simulink model "FIC_hapticControl"  (R2019b)
settings: Solver=VariableStepAuto  StartTime=0.0  StopTime=inf  FixedStep=0.00001
model workspace: external: MATLAB File /home/sydney/Desktop/matlab/simulink/SimpImpCheck/Assembly1_DataFile.m (data not in the file)
undefined symbols (not defined in the file or in its folder): smiData, X, Y, Z
libraries: sm_lib x21, nesl_utility x17, fl_lib x16, ee_lib x3
(part 2 of 2)

== matlab function FIC_hapticControl/Subsystem/MATLAB Function1 ==
  data: dxd input; Xd input; Fdes input; Wmax input; x0 input; xb input; K0 input; F input; DXd output; Wmax output; x0 output; xb output; K0 output; X input
function [DXd,Wmax,x0,xb,K0] = FICDx(dxd,Xd,Fdes,Wmax,x0,xb,K0, F,X)
% b damping - /20?
haptic=false;
if haptic
b=(xb-x0)/20;
% K0 Stiffness 
if K0>=(Wmax/x0)
    % Wmax - max torque/wrench
   K0=(Wmax/x0);
end

% Force = stiffness * displacement for the end effector? last section?
% About the spring section? B and 0?
F0=K0*x0;
% end effector desired position derivative - end effector desired velocity. 
% 
dx0d=Fdes/K0;
%When desired linear reaches 1% of end effector desired velocity 
dx0=0.01*dx0d;
% Force currently being applied is not equal to desired force
% haptic search of contact
if F~=Fdes && F~= 0
    % if current position is less than desired position
    if abs(X)<=abs(Xd)
        % Velocity = desired position + dx0d? what is this x0d
        DXd=Xd+dx0d;
    else
        % change in x = (Fdesired - currentF) * 0.01 * desired pose linear region/ desired
        % force. 
        dx=(Fdes-F)*dx0/Fdes;
        % Desired Pose = desired pose + a small change in desired pose 
        DXd=dxd+dx;
    end
else
    DXd=dxd;  
end
else
    DXd=Xd;
end

end







% if F~=Fdes
%     % %          if abs(Fdes)<=F0
%     % %              DXd=Xd+(X-Xd)*Fdes/((X-Xd)*K0+(F-Fdes));
%     if F~=0
%         DXdf=((X-Xd)*Fdes)/(F);
%         if DXdf>xb
%             DXd=Fdes/K0+sign(Fdes)*xb;
%         else
%             DXd=Fdes/K0-((X-Xd)*Fdes)/(F);
%         end
%     else
%         DXd=Fdes/K0+dxd;
%     end
%     % % else
%     % %     DXd=Xd+Wmax/((F-Wmax)/(X-Xd));
%     % % end
%     if DXd>xb
%         DXd=xb;
%     end
% else
%     DXd=dxd;
% end

% 
% function [DXd,Wmax,x0,xb,K0] = FICDx(dxd,Xd,Fdes,Wmax,x0,xb,K0,F,X)
% % b damping - /20?
% b=(xb-x0)/20;
% % K0 Stiffness 
% if K0>=(Wmax/x0)
%     % Wmax - max torque/wrench
%    K0=(Wmax/x0);
% end
% 
% % Force = stiffness * displacement for the end effector? last section?
% % About the spring section? B and 0?
% F0=K0*x0;
% % end effector desired position derivative - end effector desired velocity. 
% % 
% dx0d=Fdes/K0;
% % dividing desired by 100?
% dx0=0.01*dx0d;
% % Force currently being applied is not equal to desired force
% if F~=Fdes
%     % if current position is less than desired position
%     if abs(X)<=abs(Xd)
%         % Velocity = desired position + 
%         DXd=Xd+dx0d;
%     else
%         %DXd=dxd+sign(Fdes-F)*dx;
%         dx=(Fdes-F)*dx0/Fdes;
%         DXd=dxd+dx;
% 
%     end
% else
%     DXd=dxd;  
% end
% end

== matlab function FIC_hapticControl/Subsystem1/MATLAB Function ==
  data: xmax output; Xmax input; F output; dx input; x input; Wmax input; x0 input; xb input; K0 input
function [xmax,F]=fractalImpedenceControlFc(Xmax,dx,x,Wmax,x0,xb,K0)
b=(xb-x0)/20;
if sign(x)==-sign(dx) || abs(dx)<10^(-4)
    xmax=x;
    AbsErr=abs(x);
    if AbsErr<x0
        F=K0*x;
    else
        F=sign(x)*((1-exp(-abs(AbsErr - x0)./b)).*...
            (Wmax - K0.*x0)+K0.*x0);
    end
else
    if Xmax==0 || x>Xmax
        xmax=x;
    else
        xmax=Xmax;
        
    end
    xmid=xmax/2;
    AbsXmax=abs(xmax);
    if AbsXmax<x0
        Fmax=K0*xmax;
    else
        Fmax=sign(xmax)*((1-exp(-abs(AbsXmax - x0)./b)).*...
            (Wmax - K0.*x0)+K0.*x0);
    end
    Kout=Fmax/abs(xmid);
    F=-Kout*(xmid-x);
end

end

== matlab function FIC_hapticControl/MATLAB Function5 ==
  data: angles input; xPos output; dimensions input; yPos output; zPos output
function [xPos, yPos, zPos]  = FK(angles, dimensions)

ang1 = angles(1);
ang2 = angles(2);
ang3 = angles(3);
L1 = dimensions(1);
L2 = dimensions(2);
L3 = dimensions(3);

xPos = (L1*cos(ang1) + L2*cos(ang1 + ang2) + L3*cos(ang1 + ang2 + ang3));
yPos = (L1*sin(ang1) + L2*sin(ang1 + ang2) + L3*sin(ang1 + ang2 + ang3));
zPos = 0;

== matlab function FIC_hapticControl/Subsystem1/MATLAB Function1 ==
  data: dxd input; Xd input; Fdes input; Wmax input; x0 input; xb input; K0 input; F input; DXd output; Wmax output; x0 output; xb output; K0 output; X input
function [DXd,Wmax,x0,xb,K0] = FICDx(dxd,Xd,Fdes,Wmax,x0,xb,K0, F,X)
% b damping - /20?
haptic=false;
if haptic
b=(xb-x0)/20;
% K0 Stiffness 
if K0>=(Wmax/x0)
    % Wmax - max torque/wrench
   K0=(Wmax/x0);
end

% Force = stiffness * displacement for the end effector? last section?
% About the spring section? B and 0?
F0=K0*x0;
% end effector desired position derivative - end effector desired velocity. 
% 
dx0d=Fdes/K0;
%When desired linear reaches 1% of end effector desired velocity 
dx0=0.01*dx0d;
% Force currently being applied is not equal to desired force
% haptic search of contact
if F~=Fdes && F~= 0
    % if current position is less than desired position
    if abs(X)<=abs(Xd)
        % Velocity = desired position + dx0d? what is this x0d
        DXd=Xd+dx0d;
    else
        % change in x = (Fdesired - currentF) * 0.01 * desired pose linear region/ desired
        % force. 
        dx=(Fdes-F)*dx0/Fdes;
        % Desired Pose = desired pose + a small change in desired pose 
        DXd=dxd+dx;
    end
else
    DXd=dxd;  
end
else
    DXd=Xd;
end

end



% if F~=Fdes
%     % %          if abs(Fdes)<=F0
%     % %              DXd=Xd+(X-Xd)*Fdes/((X-Xd)*K0+(F-Fdes));
%     if F~=0
%         DXdf=((X-Xd)*Fdes)/(F);
%         if DXdf>xb
%             DXd=Fdes/K0+sign(Fdes)*xb;
%         else
%             DXd=Fdes/K0-((X-Xd)*Fdes)/(F);
%         end
%     else
%         DXd=Fdes/K0+dxd;
%     end
%     % % else
%     % %     DXd=Xd+Wmax/((F-Wmax)/(X-Xd));
%     % % end
%     if DXd>xb
%         DXd=xb;
%     end
% else
%     DXd=dxd;
% end

% 
% function [DXd,Wmax,x0,xb,K0] = FICDx(dxd,Xd,Fdes,Wmax,x0,xb,K0,F,X)
% % b damping - /20?
% b=(xb-x0)/20;
% % K0 Stiffness 
% if K0>=(Wmax/x0)
%     % Wmax - max torque/wrench
%    K0=(Wmax/x0);
% end
% 
% % Force = stiffness * displacement for the end effector? last section?
% % About the spring section? B and 0?
% F0=K0*x0;
% % end effector desired position derivative - end effector desired velocity. 
% % 
% dx0d=Fdes/K0;
% % dividing desired by 100?
% dx0=0.01*dx0d;
% % Force currently being applied is not equal to desired force
% if F~=Fdes
%     % if current position is less than desired position
%     if abs(X)<=abs(Xd)
%         % Velocity = desired position + 
%         DXd=Xd+dx0d;
%     else
%         %DXd=dxd+sign(Fdes-F)*dx;
%         dx=(Fdes-F)*dx0/Fdes;
%         DXd=dxd+dx;
% 
%     end
% else
%     DXd=dxd;  
% end
% end

== matlab function FIC_hapticControl/Subsystem2/MATLAB Function ==
  data: xmax output; Xmax input; F output; dx input; x input; Wmax input; x0 input; xb input; K0 input
function [xmax,F]=fractalImpedenceControlFc(Xmax,dx,x,Wmax,x0,xb,K0)
b=(xb-x0)/20;
if sign(x)==-sign(dx) || dx==0
    xmax=x;
    AbsErr=abs(x);
    if AbsErr<x0
        F=K0*x;
    else
        F=sign(x)*((1-exp(-abs(AbsErr - x0)./b)).*...
            (Wmax - K0.*x0)+K0.*x0);
    end
else
    if Xmax==0 || x>Xmax
        xmax=x;
    else
        xmax=Xmax;
        
    end
    xmid=xmax/2;
    AbsXmax=abs(xmax);
    if AbsXmax<x0
        Fmax=K0*xmax;
    else
        Fmax=sign(xmax)*((1-exp(-abs(AbsXmax - x0)./b)).*...
            (Wmax - K0.*x0)+K0.*x0);
    end
    Kout=Fmax/abs(xmid);
    F=-Kout*(xmid-x);
end

end

== matlab function FIC_hapticControl/Subsystem2/MATLAB Function1 ==
  data: dxd input; Xd input; Fdes input; Wmax input; x0 input; xb input; K0 input; F input; DXd output; Wmax output; x0 output; xb output; K0 output; X input
function [DXd,Wmax,x0,xb,K0] = FICDx(dxd,Xd,Fdes,Wmax,x0,xb,K0, F,X)
% b damping - /20?
haptic=false;
if haptic
b=(xb-x0)/20;
% K0 Stiffness 
if K0>=(Wmax/x0)
    % Wmax - max torque/wrench
   K0=(Wmax/x0);
end

% Force = stiffness * displacement for the end effector? last section?
% About the spring section? B and 0?
F0=K0*x0;
% end effector desired position derivative - end effector desired velocity. 
% 
dx0d=Fdes/K0;
%When desired linear reaches 1% of end effector desired velocity 
dx0=0.01*dx0d;
% Force currently being applied is not equal to desired force
% haptic search of contact
if F~=Fdes && F~= 0
    % if current position is less than desired position
    if abs(X)<=abs(Xd)
        % Velocity = desired position + dx0d? what is this x0d
        DXd=Xd+dx0d;
    else
        % change in x = (Fdesired - currentF) * 0.01 * desired pose linear region/ desired
        % force. 
        dx=(Fdes-F)*dx0/Fdes;
        % Desired Pose = desired pose + a small change in desired pose 
        DXd=dxd+dx;
    end
else
    DXd=dxd;  
end
else
    DXd=Xd;
end

end






% if F~=Fdes
%     % %          if abs(Fdes)<=F0
%     % %              DXd=Xd+(X-Xd)*Fdes/((X-Xd)*K0+(F-Fdes));
%     if F~=0
%         DXdf=((X-Xd)*Fdes)/(F);
%         if DXdf>xb
%             DXd=Fdes/K0+sign(Fdes)*xb;
%         else
%             DXd=Fdes/K0-((X-Xd)*Fdes)/(F);
%         end
%     else
%         DXd=Fdes/K0+dxd;
%     end
%     % % else
%     % %     DXd=Xd+Wmax/((F-Wmax)/(X-Xd));
%     % % end
%     if DXd>xb
%         DXd=xb;
%     end
% else
%     DXd=dxd;
% end

% 
% function [DXd,Wmax,x0,xb,K0] = FICDx(dxd,Xd,Fdes,Wmax,x0,xb,K0,F,X)
% % b damping - /20?
% b=(xb-x0)/20;
% % K0 Stiffness 
% if K0>=(Wmax/x0)
%     % Wmax - max torque/wrench
%    K0=(Wmax/x0);
% end
% 
% % Force = stiffness * displacement for the end effector? last section?
% % About the spring section? B and 0?
% F0=K0*x0;
% % end effector desired position derivative - end effector desired velocity. 
% % 
% dx0d=Fdes/K0;
% % dividing desired by 100?
% dx0=0.01*dx0d;
% % Force currently being applied is not equal to desired force
% if F~=Fdes
%     % if current position is less than desired position
%     if abs(X)<=abs(Xd)
%         % Velocity = desired position + 
%         DXd=Xd+dx0d;
%     else
%         %DXd=dxd+sign(Fdes-F)*dx;
%         dx=(Fdes-F)*dx0/Fdes;
%         DXd=dxd+dx;
% 
%     end
% else
%     DXd=dxd;  
% end
% end
